simulink model "intelligent_comfort_monitor"  (R2025b)
settings: Solver=VariableStepAuto  StartTime=0.0  StopTime=50  RelTol=1e-3
libraries: simulink x3
settings Model: Creator=Jmanu  LastModifiedBy=Jmanu

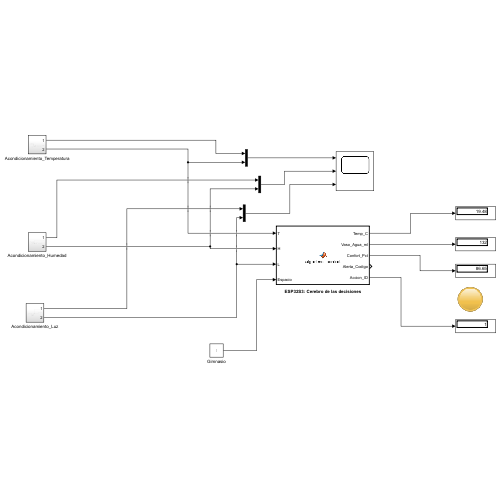
[thumbnail: Simulink's stored preview of the top-level diagram]
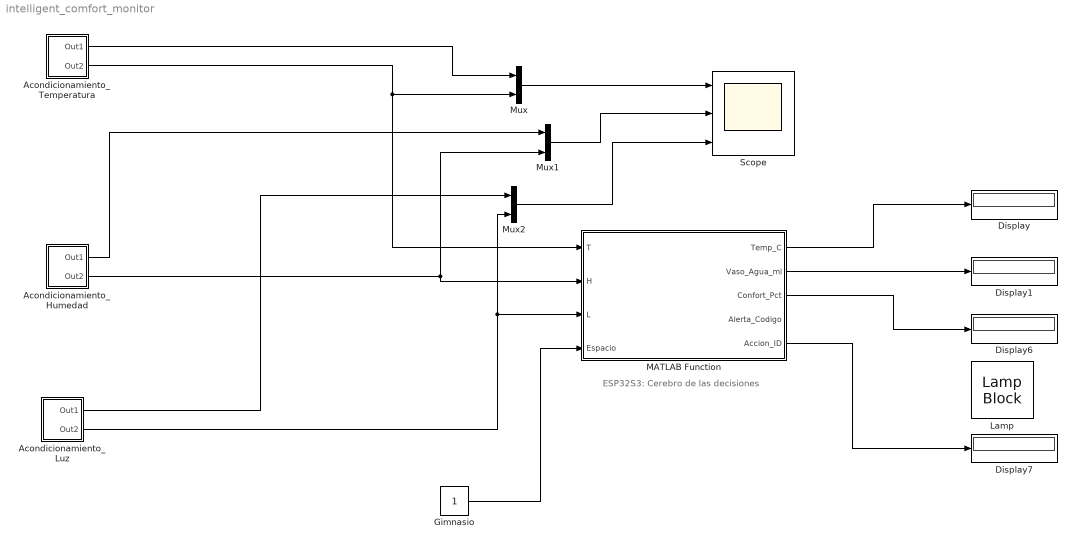
== system intelligent_comfort_monitor ==
  note: ESP32S3: Cerebro de las decisiones
  Acondicionamiento_Humedad : Subsystem
  Acondicionamiento_Luz : Subsystem
  Acondicionamiento_Temperatura : Subsystem
  Display{,1,6..7} (4 alike) : Display
  Gimnasio : Constant
  Lamp : LampBlock  LabelPosition=Hide  DefaultColor=[192.0, 192.0, 192.0]
  MATLAB Function : MATLAB Function  TreatAsAtomicUnit=on
  Mux : Mux  Inputs=2
  Mux1 : Mux  Inputs=2
  Mux2 : Mux  Inputs=2
  Scope : Scope  NumInputPorts=3
      settings: ActiveDisplayYMinimum=18.260187413599461  ActiveDisplayYMaximum=20.540059468599321
  wires:
  MATLAB Function/1(Temp_C) -> Display/1
  MATLAB Function/2(Vaso_Agua_ml) -> Display1/1
  MATLAB Function/3(Confort_Pct) -> Display6/1
  MATLAB Function/5(Accion_ID) -> Display7/1
  Gimnasio/1 -> MATLAB Function/4(Espacio)
  Mux/1 -> Scope/1
  Mux1/1 -> Scope/2
  Mux2/1 -> Scope/3
  Acondicionamiento_Temperatura/2(Out2) -> MATLAB Function/1(T), Mux/2
  Acondicionamiento_Temperatura/1(Out1) -> Mux/1
  Acondicionamiento_Humedad/2(Out2) -> Mux1/2, MATLAB Function/2(H)
  Acondicionamiento_Humedad/1(Out1) -> Mux1/1
  Acondicionamiento_Luz/2(Out2) -> Mux2/2, MATLAB Function/3(L)
  Acondicionamiento_Luz/1(Out1) -> Mux2/1

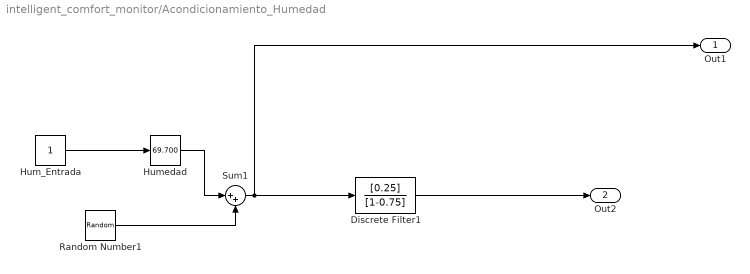
== system intelligent_comfort_monitor/Acondicionamiento_Humedad ==
  Discrete Filter1 : DiscreteFilter  Numerator=[0.25]  Denominator=[1-0.75]
  Hum_Entrada : Constant
  Humedad : simulink/Math Operations/Slider Gain  gain=69.700  low=20  high=90
  Random Number1 : RandomNumber  Variance=4  Seed=1  SampleTime=0.1
  Sum1 : Sum  Inputs=|++
  Out1 : Outport
  Out2 : Outport  Port=2
  wires:
  Hum_Entrada/1 -> Humedad/1
  Humedad/1 -> Sum1/1
  Random Number1/1 -> Sum1/2
  Sum1/1 -> Out1/1, Discrete Filter1/1
  Discrete Filter1/1 -> Out2/1

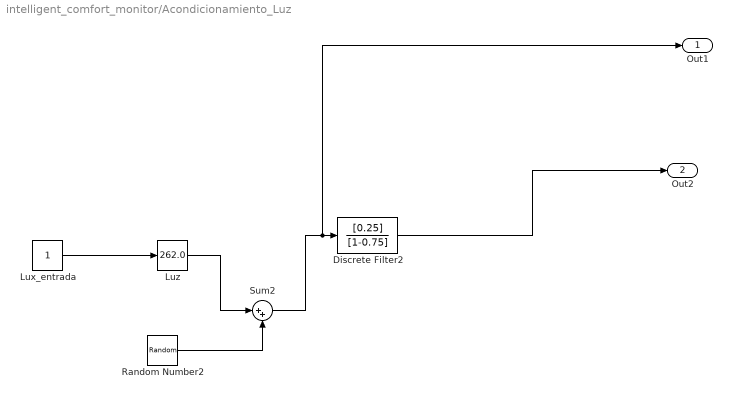
== system intelligent_comfort_monitor/Acondicionamiento_Luz ==
  Discrete Filter2 : DiscreteFilter  Numerator=[0.25]  Denominator=[1-0.75]
  Lux_entrada : Constant
  Luz : simulink/Math Operations/Slider Gain  gain=262.0  low=100  high=1000
  Random Number2 : RandomNumber  Variance=64  Seed=2  SampleTime=0.1
  Sum2 : Sum  Inputs=|++
  Out1 : Outport
  Out2 : Outport  Port=2
  wires:
  Luz/1 -> Sum2/1
  Discrete Filter2/1 -> Out2/1
  Lux_entrada/1 -> Luz/1
  Random Number2/1 -> Sum2/2
  Sum2/1 -> Out1/1, Discrete Filter2/1

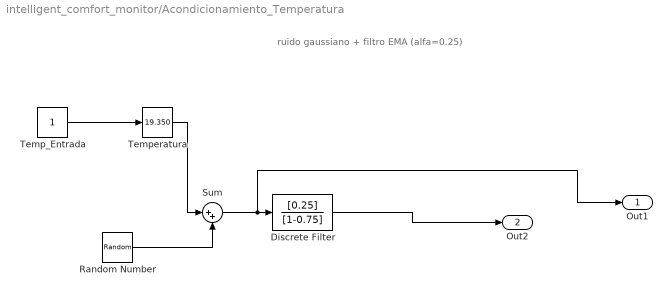
== system intelligent_comfort_monitor/Acondicionamiento_Temperatura ==
  note: ruido gaussiano + filtro EMA (alfa=0.25)
  Discrete Filter : DiscreteFilter  Numerator=[0.25]  Denominator=[1-0.75]
  Random Number : RandomNumber  Variance=0.09  SampleTime=0.1
  Sum : Sum  Inputs=|++
  Temp_Entrada : Constant
  Temperatura : simulink/Math Operations/Slider Gain  gain=19.350  low=5  high=40
  Out1 : Outport
  Out2 : Outport  Port=2
  wires:
  Random Number/1 -> Sum/2
  Temp_Entrada/1 -> Temperatura/1
  Sum/1 -> Out1/1, Discrete Filter/1
  Discrete Filter/1 -> Out2/1
  Temperatura/1 -> Sum/1

== matlab function intelligent_comfort_monitor/MATLAB Function ==
  data: T input; Temp_C output; Vaso_Agua_ml output; Confort_Pct output; H input; L input; Espacio input; Alerta_Codigo output; Accion_ID output
function [Temp_C, Vaso_Agua_ml, Confort_Pct, Alerta_Codigo, Accion_ID] = algoritmo_confort(T, H, L, Espacio)
% ALGORITMO INTELLIGENT COMFORT MONITOR - EDICIÓN B2B
%
% Entradas:
%   T: Temperatura actual (°C)
%   H: Humedad Relativa (%)
%   L: Iluminación / Radiación Solar (Lux)
%   Espacio: 1 = Gimnasio, 2 = Cancha Sintética, 3 = Skatepark
%
% Salidas:
%   Temp_C: Temperatura en °C
%   Vaso_Agua_ml: Mililitros de agua recomendados cada 20 min
%   Confort_Pct: Porcentaje óptimo para entrenar (0 a 100%)
%   Alerta_Codigo: Estado de semáforo para bloque Lamp (1=Verde, 2=Amarillo, 3=Rojo)
%   Accion_ID: ID de acción extra/creativa por tasa de sudor

    % 1. Salida directa de temperatura
    Temp_C = T;

    % 2. Factores del Espacio (Sensación térmica y radiación por superficie)
    switch Espacio
        case 1 % Gimnasio Cerrado
            Factor_Actividad = 0.85; 
            Radiacion_Extra  = 0.0;
            
        case 2 % Cancha Sintética (Calor radiante del caucho sintético)
            Factor_Actividad = 1.25; 
            Radiacion_Extra  = (L > 500) * ((L - 500) * 0.005);
            
        case 3 % Skatepark (Radiación reflejada en concreto)
            Factor_Actividad = 1.05; 
            Radiacion_Extra  = (L > 300) * ((L - 300) * 0.004);
            
        otherwise
            Factor_Actividad = 0.85;
            Radiacion_Extra  = 0.0;
    end

    T_efectiva = T + (0.05 * H) + Radiacion_Extra;

    % 3. Cálculo de Confort Ambiental Global (%)
    Penalizacion = abs(T_efectiva - 21) * 3.5 + abs(H - 50) * 0.4;
    Confort_Pct  = max(0, min(100, 100 - Penalizacion));

    % 4. LÓGICA DE SEMÁFORO MULTIVARIABLE (Salida Escalar para el Lamp)
    % Evaluación de rangos óptimos individuales
    es_temp_opt = (T >= 18.0) && (T <= 24.0);
    es_hum_opt  = (H >= 40.0) && (H <= 60.0);
    es_lux_opt  = (L <= 600);

    % Evaluación de límites críticos
    es_temp_crit = (T > 30.0);
    es_hum_crit  = (H > 75.0);
    es_lux_crit  = (L > 900);

    if es_temp_opt && es_hum_opt && es_lux_opt
        Alerta_Codigo = 1;     % VERDE: Las 3 variables están en su rango ideal
    elseif es_temp_crit || es_hum_crit || es_lux_crit
        Alerta_Codigo = 3;     % ROJO: Al menos una variable superó el límite crítico
    else
        Alerta_Codigo = 2;     % AMARILLO: Condición intermedia de precaución
    end

    % 5. Tasa de Sudor (L/h) y Rehidratación Sugerida (ml)
    Tasa_Sudor   = 0.4 + max(0, T_efectiva - 20) * 0.04 * Factor_Actividad;
    Vaso_Agua_ml = round((Tasa_Sudor * 1000 * 0.80) / 3);

    % 6. ACCIONES CREATIVAS ADICIONALES (Según Tasa_Sudor)
    if Tasa_Sudor < 0.7
        Accion_ID = 1; % "Condición Top: Apto para récords y máxima potencia."
    elseif Tasa_Sudor < 1.2
        Accion_ID = 2; % "Perdiendo grip: Aplica magnesio en manos o seca suelas."
    elseif Tasa_Sudor < 1.8
        Accion_ID = 3; % "Ropa saturada: Cambia de camiseta y consume suero/electrolitos."
    else
        Accion_ID = 4; % "Riesgo de calambre: Reduce la carga un 30% e ir a la sombra."
    end
end
